simulink model "LLL0000000"  (R2020b)
settings: Solver=VariableStepAuto  StartTime=0.0  StopTime=10.0  RelTol=1e-3
undefined symbols (not defined in the file or in its folder): P_LCS_DesLineA0FilterTime, P_LCS_DyFilterTime
settings Model: Creator=GW00216231  LastModifiedBy=GW00216231

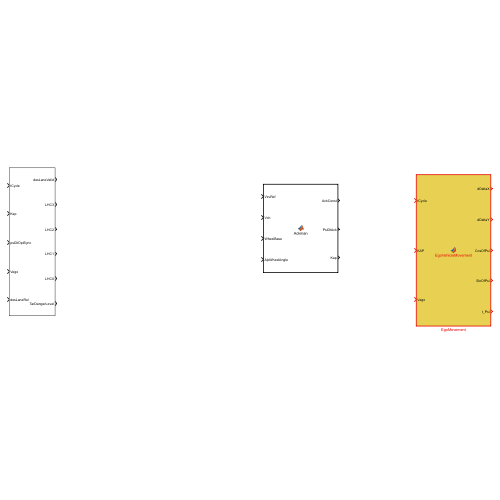
[thumbnail: Simulink's stored preview of the top-level diagram]
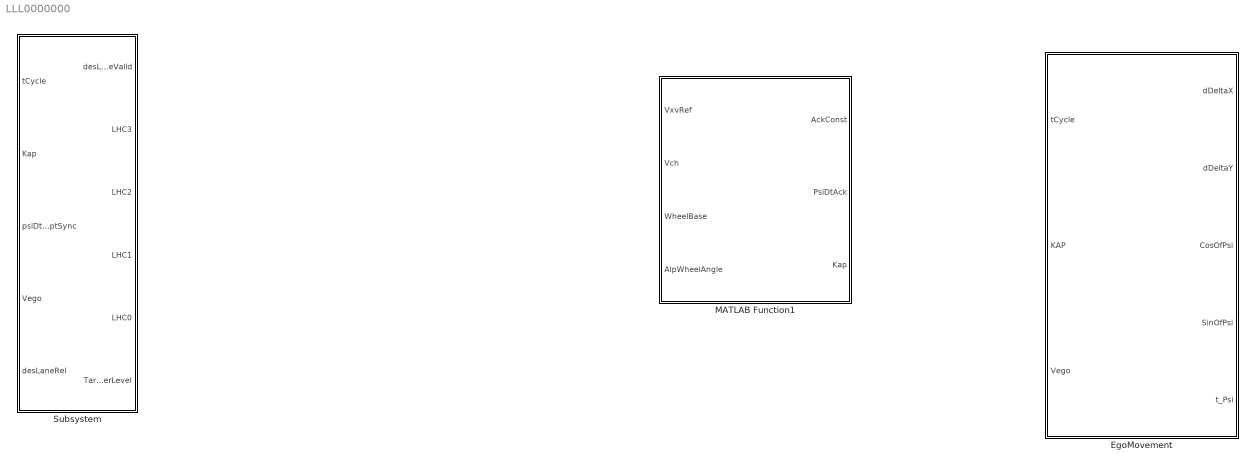
== system LLL0000000 ==
  EgoMovement : MATLAB Function  TreatAsAtomicUnit=on
  MATLAB Function1 : MATLAB Function  TreatAsAtomicUnit=on
  Subsystem : Subsystem

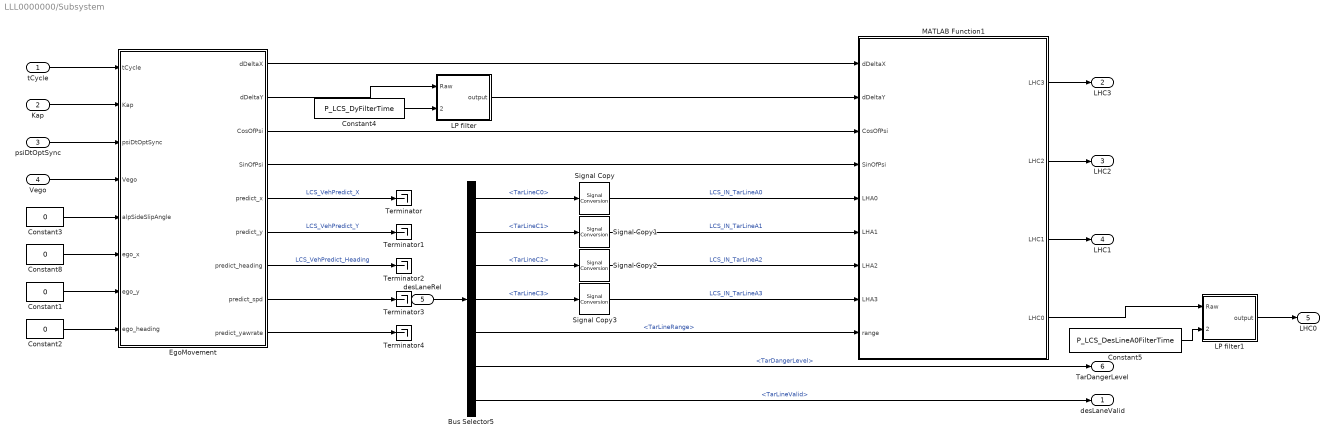
== system LLL0000000/Subsystem ==
  tCycle : Inport
  Kap : Inport  Port=2
  psiDtOptSync : Inport  Port=3
  Vego : Inport  Port=4
  desLaneRel : Inport  Port=5
  Bus Selector5 : BusSelector  OutputSignals=TarLineC0,TarLineC1,TarLineC2,TarLineC3,TarLineRange,TarDangerLevel,TarLineValid
  Constant{1..3,8} (4 alike) : Constant  Value=0  OutDataTypeStr=single
  Constant4 : Constant  Value=P_LCS_DyFilterTime  OutDataTypeStr=single
  Constant5 : Constant  Value=P_LCS_DesLineA0FilterTime  OutDataTypeStr=single
  EgoMovement : MATLAB Function  TreatAsAtomicUnit=on
  LP filter : Subsystem
  LP filter1 : Subsystem
  MATLAB Function1 : MATLAB Function  TreatAsAtomicUnit=on
  Signal Copy{,1..3} (4 alike) : SignalConversion  OverrideOpt=off
  Terminator{,1..4} (5 alike) : Terminator
  desLaneValid : Outport
  LHC3 : Outport  Port=2
  LHC2 : Outport  Port=3
  LHC1 : Outport  Port=4
  LHC0 : Outport  Port=5
  TarDangerLevel : Outport  Port=6
  wires:
  tCycle/1 -> EgoMovement/1(tCycle)
  Bus Selector5/4 -> Signal Copy3/1  "<TarLineC3>"
  Constant3/1 -> EgoMovement/5(alpSideSlipAngle)
  Bus Selector5/3 -> Signal Copy2/1  "<TarLineC2>"
  Bus Selector5/5 -> MATLAB Function1/9(range)  "<TarLineRange>"
  Bus Selector5/1 -> Signal Copy/1  "<TarLineC0>"
  Bus Selector5/2 -> Signal Copy1/1  "<TarLineC1>"
  MATLAB Function1/1(LHC3) -> LHC3/1
  desLaneRel/1 -> Bus Selector5/1
  EgoMovement/3(CosOfPsi) -> MATLAB Function1/3(CosOfPsi)
  EgoMovement/1(dDeltaX) -> MATLAB Function1/1(dDeltaX)
  MATLAB Function1/3(LHC1) -> LHC1/1
  EgoMovement/4(SinOfPsi) -> MATLAB Function1/4(SinOfPsi)
  EgoMovement/2(dDeltaY) -> LP filter/1(Raw)
  Kap/1 -> EgoMovement/2(Kap)
  psiDtOptSync/1 -> EgoMovement/3(psiDtOptSync)
  Vego/1 -> EgoMovement/4(Vego)
  MATLAB Function1/2(LHC2) -> LHC2/1
  MATLAB Function1/4(LHC0) -> LP filter1/1(Raw)
  EgoMovement/5(predict_x) -> Terminator/1  "LCS_VehPredict_X"
  Bus Selector5/7 -> desLaneValid/1  "<TarLineValid>"
  Bus Selector5/6 -> TarDangerLevel/1  "<TarDangerLevel>"
  Constant8/1 -> EgoMovement/6(ego_x)
  Constant1/1 -> EgoMovement/7(ego_y)
  Constant2/1 -> EgoMovement/8(ego_heading)
  EgoMovement/6(predict_y) -> Terminator1/1  "LCS_VehPredict_Y"
  EgoMovement/7(predict_heading) -> Terminator2/1  "LCS_VehPredict_Heading"
  EgoMovement/8(predict_spd) -> Terminator3/1
  EgoMovement/9(predict_yawrate) -> Terminator4/1
  Signal Copy/1 -> MATLAB Function1/5(LHA0)  "LCS_IN_TarLineA0"
  Signal Copy1/1 -> MATLAB Function1/6(LHA1)  "LCS_IN_TarLineA1"
  Signal Copy2/1 -> MATLAB Function1/7(LHA2)  "LCS_IN_TarLineA2"
  Signal Copy3/1 -> MATLAB Function1/8(LHA3)  "LCS_IN_TarLineA3"
  LP filter/1(output) -> MATLAB Function1/2(dDeltaY)
  Constant4/1 -> LP filter/2(TorqFilterTime)
  LP filter1/1(output) -> LHC0/1
  Constant5/1 -> LP filter1/2(TorqFilterTime)

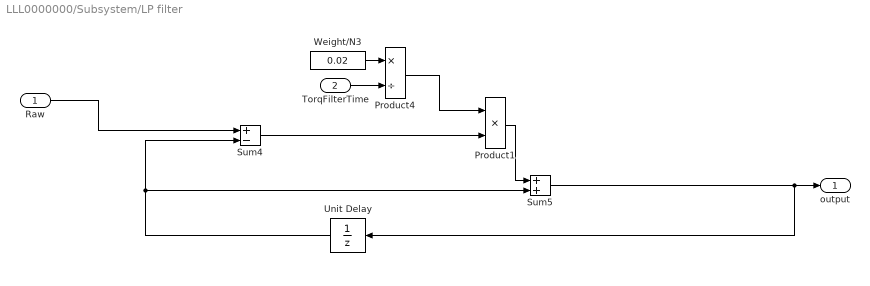
== system LLL0000000/Subsystem/LP filter ==
  Raw : Inport
  TorqFilterTime : Inport  Port=2
  Product1 : Product  RndMeth=Zero
  Product4 : Product  Inputs=*/  RndMeth=Zero
  Sum4 : Sum  Inputs=+-
  Sum5 : Sum
  Unit Delay : UnitDelay  SampleTime=-1  HasFrameUpgradeWarning=on
  Weight/N3 : Constant  Value=0.02  OutDataTypeStr=single
  output : Outport
  wires:
  TorqFilterTime/1 -> Product4/2
  Product4/1 -> Product1/1
  Weight/N3/1 -> Product4/1
  Raw/1 -> Sum4/1
  Product1/1 -> Sum5/1
  Sum4/1 -> Product1/2
  Unit Delay/1 -> Sum5/2, Sum4/2
  Sum5/1 -> output/1, Unit Delay/1

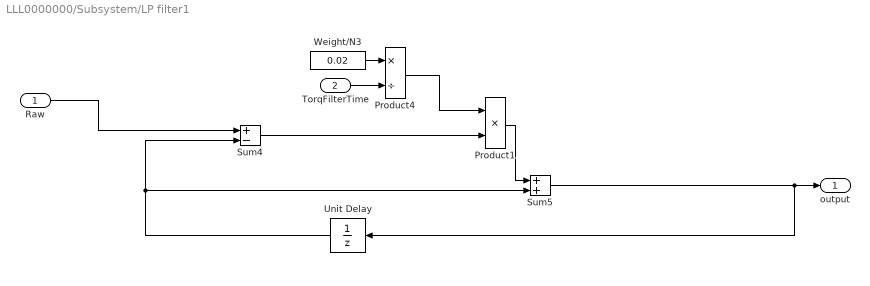
== system LLL0000000/Subsystem/LP filter1 ==
  Raw : Inport
  TorqFilterTime : Inport  Port=2
  Product1 : Product  RndMeth=Zero
  Product4 : Product  Inputs=*/  RndMeth=Zero
  Sum4 : Sum  Inputs=+-
  Sum5 : Sum
  Unit Delay : UnitDelay  SampleTime=-1  HasFrameUpgradeWarning=on
  Weight/N3 : Constant  Value=0.02  OutDataTypeStr=single
  output : Outport
  wires:
  TorqFilterTime/1 -> Product4/2
  Product4/1 -> Product1/1
  Weight/N3/1 -> Product4/1
  Raw/1 -> Sum4/1
  Product1/1 -> Sum5/1
  Sum4/1 -> Product1/2
  Unit Delay/1 -> Sum5/2, Sum4/2
  Sum5/1 -> output/1, Unit Delay/1

== matlab function LLL0000000/Subsystem/MATLAB Function1 ==
  data: dDeltaX input; dDeltaY input; CosOfPsi input; SinOfPsi input; LHA0 input; LHC3 output; LHA1 input; LHA2 input; LHA3 input; range input; LHC2 output; LHC1 output; LHC0 output
function [LHC3,LHC2,LHC1,LHC0] = fcn(dDeltaX,dDeltaY,CosOfPsi,SinOfPsi,LHA0,LHA1,LHA2,LHA3,range)

 % temp_x = [0,1/4*range,1/2*range,range];
 temp_x = [0,20,40,80];
  
 y1 = LHA0+LHA1*temp_x(1)+LHA2*temp_x(1)^2+LHA3*temp_x(1)^3;
 y2 = LHA0+LHA1*temp_x(2)+LHA2*temp_x(2)^2+LHA3*temp_x(2)^3;
 y3 = LHA0+LHA1*temp_x(3)+LHA2*temp_x(3)^2+LHA3*temp_x(3)^3;
 y4 = LHA0+LHA1*temp_x(4)+LHA2*temp_x(4)^2+LHA3*temp_x(4)^3;
 temp_y = [y1,y2,y3,y4];
 t_dx = temp_x-dDeltaX;
 t_dy = temp_y-dDeltaY;
 TmpX = t_dx*CosOfPsi+t_dy*SinOfPsi;
 TmpY = -t_dx*SinOfPsi+t_dy*CosOfPsi;
%  P = polyfit(TmpX,TmpY,3);
%  LHC3 = P(1);
%  LHC2 = P(2);
%  LHC1 = P(3);
%  LHC0 = P(4);
 [A,B,C,D] = pl(TmpX,TmpY);
 LHC3 = A;
 LHC2 = B;
 LHC1 = C;
 LHC0 = D;
end
 function [A,B,C,D] = pl(X,Y)
MatrixA = [X(1)^3,X(1)^2,X(1),1;...
           X(2)^3,X(2)^2,X(2),1;...
           X(3)^3,X(3)^2,X(3),1;...
           X(4)^3,X(4)^2,X(4),1];
MatrixB = [Y(1);Y(2);Y(3);Y(4)];
if det(MatrixA)==0
    A=cast(0,class(X(1)));
    B=cast(0,class(X(1)));
    C=cast(0,class(X(1)));
    D=cast(0,class(X(1)));
else
    P = MatrixA\MatrixB;
    A = P(1);
    B = P(2);
    C = P(3);
    D = P(4);
end
% coder.allowpcode('plain');
end

== matlab function LLL0000000/EgoMovement ==
  data: dDeltaX output single size=1; dDeltaY output single size=1; tCycle input single; CosOfPsi output single size=1; KAP input single; Vego input single; SinOfPsi output single size=1; t_Psi output
function [dDeltaX,dDeltaY,CosOfPsi,SinOfPsi,t_Psi] = EgoVehicleMovement(tCycle,KAP,Vego)
%#codegen
dDeltaX = single(0);
dDeltaY = single(0);
t_Psi = single(0);
for i = 1:(length(KAP)-1) % KAP 从最早时间开始排列
    Kap = KAP(i);
    if Kap==0
        dDeltaX = dDeltaX + Vego(i)*tCycle;
        dDeltaY = dDeltaY + single(0);
        CosOfPsi = single(1);
        SinOfPsi = single(0);
    else
        d_Psi = Kap*Vego(i)*tCycle;
        SinOfPsi = sin(d_Psi);
        CosOfPsi = cos(d_Psi);
        dDeltaX = dDeltaX + SinOfPsi/Kap;
        dDeltaY = dDeltaY + 2*(sin(d_Psi/2)*sin(d_Psi/2))/Kap;
        t_Psi = t_Psi + d_Psi;
    end
end

== matlab function LLL0000000/MATLAB Function1 ==
  data: VxvRef input; AckConst output; Vch input; WheelBase input; AlpWheelAngle input; PsiDtAck output; Kap output
function [AckConst,PsiDtAck,Kap] = Ackman(VxvRef,Vch,WheelBase,AlpWheelAngle)
%#codegen
AckConst = single(zeros(1,1));
PsiDtAck = single(zeros(length(AlpWheelAngle),1));
Kap = single(zeros(length(AlpWheelAngle),1));
for i = 1:length(AlpWheelAngle)
    if VxvRef(i,1)==uint8(0)%转换常数数据类型
        PsiDtAck(i,1) = single(0);%转换常数数据类型
        AckConst = single(1);%转换常数数据类型
    else
        AckConst = min((single(1)+VxvRef(i,1)*VxvRef(i,1)/(Vch*Vch))*WheelBase/VxvRef(i,1),single(32767));%转换常数数据类型
        PsiDtAck(i,1) = AlpWheelAngle(i,1)/AckConst;
    end
    Kap(i,1) =  PsiDtAck(i,1)/max(VxvRef(i,1),0.5);
end
end

== matlab function LLL0000000/Subsystem/EgoMovement ==
  data: dDeltaX output single size=1; dDeltaY output single size=1; tCycle input single size=1; CosOfPsi output single size=1; Kap input single size=1; psiDtOptSync input single size=1; Vego input single size=1; alpSideSlipAngle input single size=1; SinOfPsi output single size=1; ego_x input; ego_y input; ego_heading input; predict_x output; predict_y output; predict_heading output; predict_spd output; predict_yawrate output
function [dDeltaX,dDeltaY,CosOfPsi,SinOfPsi,predict_x,predict_y,predict_heading,predict_spd,predict_yawrate] = EgoVehicleMovement(tCycle,Kap,psiDtOptSync,Vego,alpSideSlipAngle,ego_x,ego_y,ego_heading)
%#codegen
if Kap==0
    dDeltaX = Vego*tCycle;
    dDeltaY = single(0);
    CosOfPsi = single(1);
    SinOfPsi = single(0);
    t_Psi = single(0);
else
    t_kap = Kap;
    if ((Kap>0.125)||(Kap<-0.125))&&(Vego>1)
        t_kapPsiDtSync = psiDtOptSync/Vego;    %实际计算的曲率
        if abs(t_kapPsiDtSync)>abs(Kap)          
            t_kap = t_kapPsiDtSync;
        end
    end
    t_Psi = t_kap*Vego*tCycle;
    SinOfPsi = sin(t_Psi);
    CosOfPsi = cos(t_Psi);
    t_dDeltaXTemp = SinOfPsi/t_kap;
    t_dDeltaYTemp = 2*(sin(t_Psi/2)*sin(t_Psi/2))/t_kap;
    dDeltaX = cos(alpSideSlipAngle)*t_dDeltaXTemp - sin(alpSideSlipAngle)*t_dDeltaYTemp;
    dDeltaY = sin(alpSideSlipAngle)*t_dDeltaXTemp + cos(alpSideSlipAngle)*t_dDeltaYTemp;
end
predict_x = ego_x + dDeltaX;
predict_y = ego_y + dDeltaY;
predict_heading = ego_heading + t_Psi;
predict_spd = Vego;
predict_yawrate = psiDtOptSync;
end
